simulink model "Three_phase_bridge_LR1"  (Simulink 6.1)
settings: Solver=ode23tb  StartTime=0.0  StopTime=0.1499  MaxStep=1e-4  RelTol=1e-3  AbsTol=.01
libraries: powerlib x15
settings Model: LastModifiedBy=ThinkPad
settings DebuggingCC: SolverPrmCheckMsg=warning

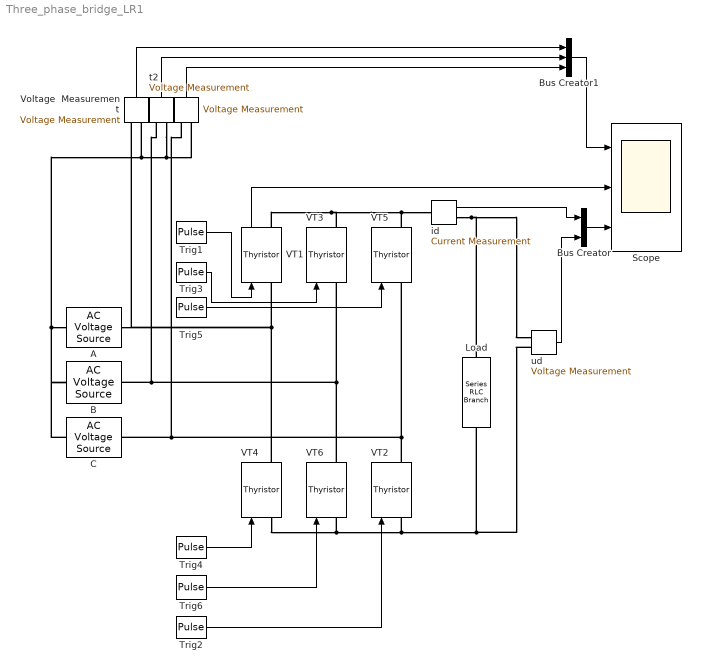
== system Three_phase_bridge_LR1 ==
  "   " : powerlib/Measurements/Voltage Measurement  Orientation=up  PhasorSimulation=off  OutputType=Complex  PSBequivalent=0
  A : powerlib/Electrical Sources/AC Voltage Source  Amplitude=100  Phase=30  Frequency=50  SampleTime=0  Measurements=None
  B : powerlib/Electrical Sources/AC Voltage Source  Amplitude=100  Phase=-90  Frequency=50  SampleTime=0  Measurements=None
  Bus Creator : BusCreator  DialogController=Simulink.DDGSource_Bus  Inputs=2
  Bus Creator1 : BusCreator  DialogController=Simulink.DDGSource_Bus  Inputs=3
  C : powerlib/Electrical Sources/AC Voltage Source  Amplitude=100  Phase=-210  Frequency=50  SampleTime=0  Measurements=None
  Load : powerlib/Elements/Series RLC Branch  Orientation=down  PhysicalDomain=powersysdomain  SubClassName=unknown  LeftPortType=p1  RightPortType=p1  LConnTagsString=__new0  RConnTagsString=__new0  Resistance=2  Inductance=0.01  Capacitance=inf  Measurements=None
  Scope : Scope  NumInputPorts=3
      settings: TimeRange=0.05  YMin=-100~-200~-200  YMax=100~200~200  Decimation=5  SampleInput=on  SampleTime=1e-4
  Trig1 : DiscretePulseGenerator  PulseType=Time based  Amplitude=10  Period=0.02  PulseWidth=20
  Trig2 : DiscretePulseGenerator  PulseType=Time based  Amplitude=10  Period=0.02  PulseWidth=20  PhaseDelay=0.00333
  Trig3 : DiscretePulseGenerator  PulseType=Time based  Amplitude=10  Period=0.02  PulseWidth=20  PhaseDelay=0.00667
  Trig4 : DiscretePulseGenerator  PulseType=Time based  Amplitude=10  Period=0.02  PulseWidth=20  PhaseDelay=0.01
  Trig5 : DiscretePulseGenerator  PulseType=Time based  Amplitude=10  Period=0.02  PulseWidth=20  PhaseDelay=0.01333
  Trig6 : DiscretePulseGenerator  PulseType=Time based  Amplitude=10  Period=0.02  PulseWidth=20  PhaseDelay=0.01667
  VT{1..6} (6 alike) : powerlib/Power Electronics/Thyristor  Orientation=up  Ron=0.01  Lon=0  Vf=0.8  IC=0  Rs=1000  Cs=100e-9  Measurements=on
  Voltage  Measurement : powerlib/Measurements/Voltage Measurement  Orientation=up  PhasorSimulation=off  OutputType=Complex  PSBequivalent=0
  id : powerlib/Measurements/Current Measurement  PhasorSimulation=off  OutputType=Complex  PSBequivalent=0
  t2 : powerlib/Measurements/Voltage Measurement  Orientation=up  PhasorSimulation=off  OutputType=Complex  PSBequivalent=0
  ud : powerlib/Measurements/Voltage Measurement  PhasorSimulation=off  OutputType=Complex  PSBequivalent=0
  wires:
  VT1/1 -> Scope/2
  ud/1 -> Bus Creator/2
  Bus Creator/1 -> Scope/3
  id/1 -> Bus Creator/1
  Bus Creator1/1 -> Scope/1
  Voltage  Measurement/1 -> Bus Creator1/1
  Trig6/1 -> VT6/1
  t2/1 -> Bus Creator1/2
  "   "/1 -> Bus Creator1/3
  Trig4/1 -> VT4/1
  Trig2/1 -> VT2/1
  Trig5/1 -> VT5/1
  Trig3/1 -> VT3/1
  Trig1/1 -> VT1/1
  connections:
  id/RConn1 -- Load/LConn1 -- ud/LConn1
  VT1/RConn1 -- id/LConn1 -- VT5/RConn1 -- VT3/RConn1
  C/LConn1 -- B/LConn1 -- A/LConn1 -- t2/LConn2 -- "   "/LConn2 -- Voltage  Measurement/LConn2
  A/RConn1 -- VT4/RConn1 -- VT1/LConn1 -- Voltage  Measurement/LConn1
  VT4/LConn1 -- ud/LConn2 -- Load/RConn1 -- VT2/LConn1 -- VT6/LConn1
  VT2/RConn1 -- VT5/LConn1 -- C/RConn1 -- "   "/LConn1
  VT6/RConn1 -- VT3/LConn1 -- B/RConn1 -- t2/LConn1
